simulink model "UniformQuantificationVoice"  (R2018b)
settings: Solver=VariableStepAuto  StartTime=0.0  StopTime=10.0  RelTol=1e-3
settings Model: Creator=Anderson  LastModifiedBy=Anderson

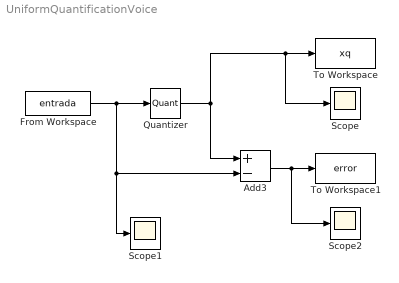
== system UniformQuantificationVoice ==
  Add3 : Sum  Inputs=+-
  From Workspace : FromWorkspace  VariableName=entrada  SampleTime=0
  Quantizer : Quantizer  QuantizationInterval=0.125
  Scope : Scope
  Scope1 : Scope
  Scope2 : Scope
  To Workspace : ToWorkspace  VariableName=xq  SaveFormat=Timeseries  SampleTime=-1
  To Workspace1 : ToWorkspace  VariableName=error  SaveFormat=Timeseries  SampleTime=-1
  wires:
  From Workspace/1 -> Scope1/1, Add3/2, Quantizer/1
  Quantizer/1 -> Add3/1, Scope/1, To Workspace/1
  Add3/1 -> Scope2/1, To Workspace1/1
